simulink model "BLOC_Engine_representation"  (R2016a)
settings: Solver=VariableStepAuto  StartTime=0.0  StopTime=10.0  RelTol=1e-3
undefined symbols (not defined in the file): hev_dt, ra_electrical_machine_speed, ra_electrical_machine_tau, ra_em_max_tq, ra_em_min_tq
libraries: simulink x1
settings Model: Creator=Florent  LastModifiedBy=Florent

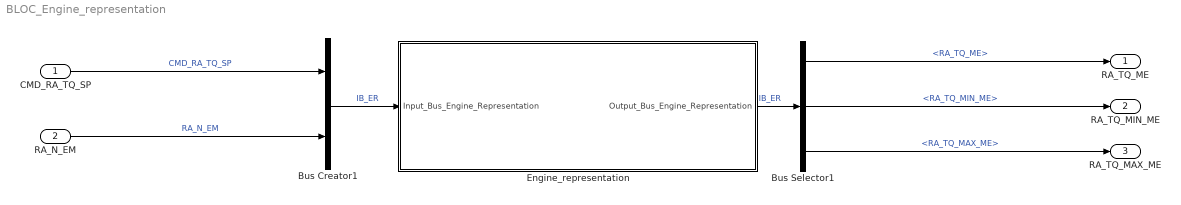
== system BLOC_Engine_representation ==
  CMD_RA_TQ_SP : Inport
  RA_N_EM : Inport  Port=2
  Bus Creator1 : BusCreator  Inputs=2
  Bus Selector1 : BusSelector  OutputSignals=RA_TQ_ME,RA_TQ_MIN_ME,RA_TQ_MAX_ME
  Engine_representation : Subsystem  TreatAsAtomicUnit=on  SystemSampleTime=hev_dt
  RA_TQ_ME : Outport
  RA_TQ_MIN_ME : Outport  Port=2
  RA_TQ_MAX_ME : Outport  Port=3
  wires:
  CMD_RA_TQ_SP/1 -> Bus Creator1/1  "CMD_RA_TQ_SP"
  RA_N_EM/1 -> Bus Creator1/2  "RA_N_EM"
  Bus Creator1/1 -> Engine_representation/1(Input_Bus_Engine_Representation)  "IB_ER"
  Engine_representation/1(Output_Bus_Engine_Representation) -> Bus Selector1/1  "IB_ER"
  Bus Selector1/2 -> RA_TQ_MIN_ME/1  "<RA_TQ_MIN_ME>"
  Bus Selector1/3 -> RA_TQ_MAX_ME/1  "<RA_TQ_MAX_ME>"
  Bus Selector1/1 -> RA_TQ_ME/1  "<RA_TQ_ME>"

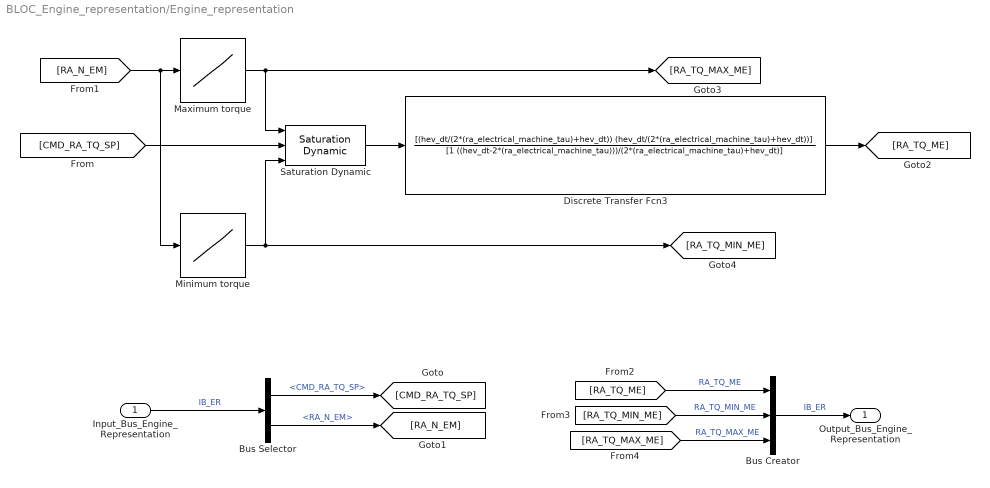
== system BLOC_Engine_representation/Engine_representation ==
  Input_Bus_Engine_Representation : Inport
  Bus Creator : BusCreator  Inputs=3
  Bus Selector : BusSelector  OutputSignals=CMD_RA_TQ_SP,RA_N_EM
  Discrete Transfer Fcn3 : DiscreteTransferFcn  Numerator=[(hev_dt/(2*(ra_electrical_machine_tau)+hev_dt)) (hev_dt/(2*(ra_electrical_machine_tau)+hev_dt))]  Denominator=[1 ((hev_dt-2*(ra_electrical_machine_tau)))/(2*(ra_electrical_machine_tau)+hev_dt)]  SampleTime=hev_dt
  Maximum torque : Lookup  InputValues=ra_electrical_machine_speed  Table=ra_em_max_tq  LookUpMeth=Interpolation-Use End Values  SampleTime=hev_dt
  Minimum torque : Lookup  InputValues=ra_electrical_machine_speed  Table=ra_em_min_tq  LookUpMeth=Interpolation-Use End Values  SampleTime=hev_dt
  Saturation Dynamic : simulink/Discontinuities/Saturation Dynamic  OutMin=[]  OutMax=[]  OutDataTypeStr=Inherit: Same as second input  OutDataType=fixdt(1, 16)  OutScaling=2^-10  DoSatur=off
  Output_Bus_Engine_Representation : Outport
  wires:
  [RA_N_EM] -> Maximum torque/1, Minimum torque/1
  Maximum torque/1 -> [RA_TQ_MAX_ME], Saturation Dynamic/1
  Minimum torque/1 -> [RA_TQ_MIN_ME], Saturation Dynamic/3
  Saturation Dynamic/1 -> Discrete Transfer Fcn3/1
  [CMD_RA_TQ_SP] -> Saturation Dynamic/2
  Discrete Transfer Fcn3/1 -> [RA_TQ_ME]
  Input_Bus_Engine_Representation/1 -> Bus Selector/1  "IB_ER"
  Bus Selector/1 -> [CMD_RA_TQ_SP]  "<CMD_RA_TQ_SP>"
  Bus Selector/2 -> [RA_N_EM]  "<RA_N_EM>"
  Bus Creator/1 -> Output_Bus_Engine_Representation/1  "IB_ER"
  [RA_TQ_ME] -> Bus Creator/1  "RA_TQ_ME"
  [RA_TQ_MIN_ME] -> Bus Creator/2  "RA_TQ_MIN_ME"
  [RA_TQ_MAX_ME] -> Bus Creator/3  "RA_TQ_MAX_ME"
